simulink model "green_joint_average_motor_square_wave_harness"  (R2023b)
settings: Solver=FixedStepDiscrete  StartTime=0.0  StopTime=GJDT_StopTime  FixedStep=GJDT_TsPlant  RelTol=1e-3
values from neighbouring files (symbols this model uses):
  GJDT_IdRef_A = single(0.0)    [setup_green_joint_current_loop_twin.m]
  GJDT_Ts = 50e-6    (= 5e-05)    [setup_green_joint_current_loop_twin.m]
  GJDT_TsPlant = 5e-6    (= 5e-06)    [setup_green_joint_current_loop_twin.m]
  GJDT_Vbus_V = single(12.0)    [setup_green_joint_current_loop_twin.m]
  motor = evalin('base', 'motor')    [sweep_green_joint_speed_loop_100us_pll_candidates.m]
  simcfg = build_sim_config(cfg, module_1620)    [design_green_joint_current_loop_with_delay.m]
undefined symbols (not defined in the file or in its folder): CurDKi, CurDKp, CurQKi, CurQKp, inverter, PiCorrectionGain, VoltageEpsilon, VoltageLimitRatio
libraries: mcbplantlib x1, autolibpmsmexterior x1
Description:
  | Visible 1 kHz current-square harness. TestSupervisor is simulation-only and is not generated controller code.
settings Model: DataDictionary=green_joint_average_motor_twin_interface.sldd  Creator=user  LastModifiedBy=user
settings DebuggingCC: ParameterPrecisionLossMsg=none

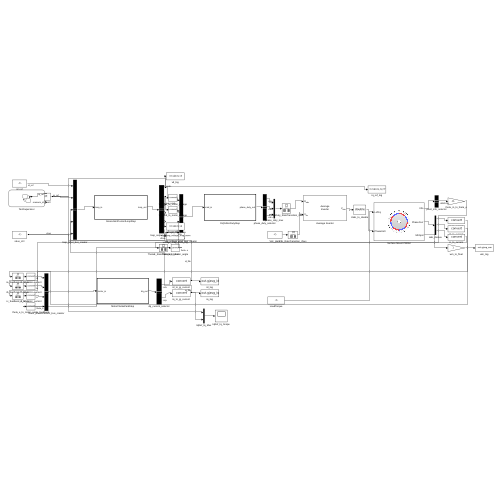
[thumbnail: Simulink's stored preview of the top-level diagram]
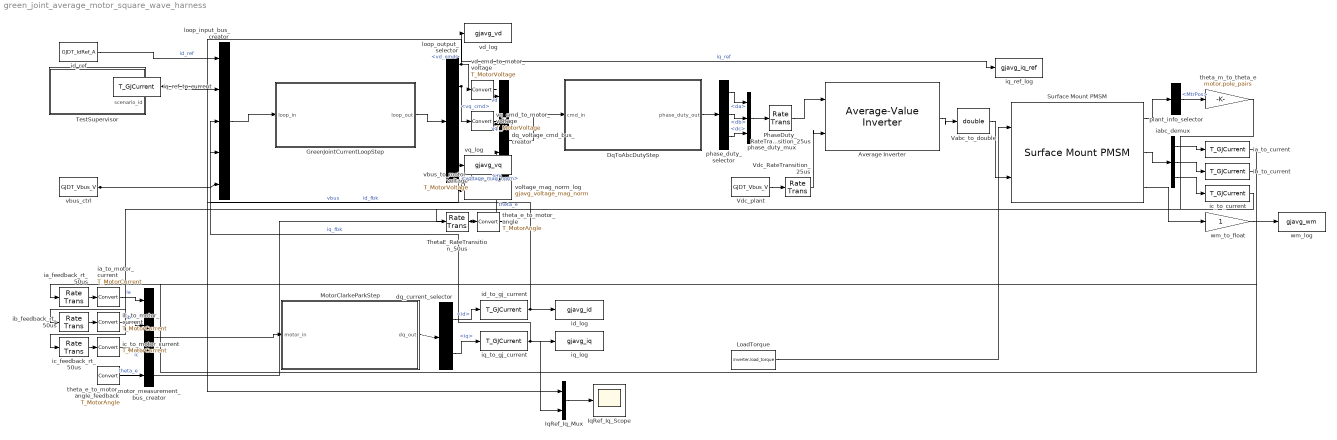
== system green_joint_average_motor_square_wave_harness ==
  Average Inverter : mcbplantlib/Average-Value Inverter
  DqToAbcDutyStep : Subsystem  TreatAsAtomicUnit=on  RTWFcnName=DqToAbcDutyStep  RTWFileName=DqToAbcDutyStep
      settings: RTWFcnNameOpts=User specified  RTWFileNameOpts=User specified
  GreenJointCurrentLoopStep : Subsystem  TreatAsAtomicUnit=on  RTWFcnName=GreenJointCurrentLoopStep  RTWFileName=GreenJointCurrentLoopStep
      settings: RTWFcnNameOpts=User specified  RTWFileNameOpts=User specified
  IqRef_Iq_Mux : Mux  Inputs=2
  IqRef_Iq_Scope : Scope
  LoadTorque : Constant  Value=inverter.load_torque  OutDataTypeStr=double  SampleTime=GJDT_TsPlant
  MotorClarkeParkStep : Subsystem  TreatAsAtomicUnit=on  RTWFcnName=MotorClarkeParkStep  RTWFileName=MotorClarkeParkStep
      settings: RTWFcnNameOpts=User specified  RTWFileNameOpts=User specified
  PhaseDuty_RateTransition_25us : RateTransition  OutPortSampleTime=GJDT_TsPlant
  Surface Mount PMSM : autolibpmsmexterior/Surface Mount PMSM  port_config=Torque  sim_type=Discrete  Ts=GJDT_TsPlant  P=motor.pole_pairs  Rs=motor.Rs  Ldq_=motor.Ld  KConstText=Permanent flux linkage constant (lambda_pm):  lambda_pm=motor.psi_f  Ke=159.9771  Kt=1.323  mechanical=[motor.J, motor.B, 0]  idq0=[0 0]  theta_init=0  omega_init=0  KConst=motor.psi_f  lambda_pm_calc=motor.psi_f  RefBlkName='autolibpmsmexterior/Surface Mount PMSM'  aMode=5  Ldq="[0.0017      0.0017]"
  TestSupervisor : Stateflow chart  TreatAsAtomicUnit=on
  ThetaE_RateTransition_50us : RateTransition  OutPortSampleTime=GJDT_Ts
  Vabc_to_double : DataTypeConversion  OutDataTypeStr=double  SaturateOnIntegerOverflow=off  RndMeth=Floor
  Vdc_RateTransition_25us : RateTransition  OutPortSampleTime=GJDT_TsPlant
  Vdc_plant : Constant  Value=GJDT_Vbus_V  OutDataTypeStr=T_GJVoltage  SampleTime=GJDT_TsPlant
  dq_current_selector : BusSelector  OutputSignals=id,iq
  dq_voltage_cmd_bus_creator : BusCreator  Inputs=4  OutDataTypeStr=Bus: open_loop_cmd_t  NonVirtualBus=on
  ia_feedback_rt_50us : RateTransition  OutPortSampleTime=GJDT_Ts
  ia_to_current : DataTypeConversion  OutDataTypeStr=T_GJCurrent  SaturateOnIntegerOverflow=off  RndMeth=Floor
  ia_to_motor_current : DataTypeConversion  OutDataTypeStr=T_MotorCurrent  SaturateOnIntegerOverflow=off  RndMeth=Floor
  iabc_demux : Demux  Outputs=3
  ib_feedback_rt_50us : RateTransition  OutPortSampleTime=GJDT_Ts
  ib_to_current : DataTypeConversion  OutDataTypeStr=T_GJCurrent  SaturateOnIntegerOverflow=off  RndMeth=Floor
  ib_to_motor_current : DataTypeConversion  OutDataTypeStr=T_MotorCurrent  SaturateOnIntegerOverflow=off  RndMeth=Floor
  ic_feedback_rt_50us : RateTransition  OutPortSampleTime=GJDT_Ts
  ic_to_current : DataTypeConversion  OutDataTypeStr=T_GJCurrent  SaturateOnIntegerOverflow=off  RndMeth=Floor
  ic_to_motor_current : DataTypeConversion  OutDataTypeStr=T_MotorCurrent  SaturateOnIntegerOverflow=off  RndMeth=Floor
  id_log : ToWorkspace  VariableName=gjavg_id  SaveFormat=Structure With Time  SampleTime=-1
  id_ref : Constant  Value=GJDT_IdRef_A  OutDataTypeStr=T_GJCurrent  SampleTime=GJDT_Ts
  id_to_gj_current : DataTypeConversion  OutDataTypeStr=T_GJCurrent  SaturateOnIntegerOverflow=off  RndMeth=Floor
  iq_log : ToWorkspace  VariableName=gjavg_iq  SaveFormat=Structure With Time  SampleTime=-1
  iq_ref_log : ToWorkspace  VariableName=gjavg_iq_ref  SaveFormat=Structure With Time  SampleTime=-1
  iq_ref_to_current : DataTypeConversion  OutDataTypeStr=T_GJCurrent  SaturateOnIntegerOverflow=off  RndMeth=Floor
  iq_to_gj_current : DataTypeConversion  OutDataTypeStr=T_GJCurrent  SaturateOnIntegerOverflow=off  RndMeth=Floor
  loop_input_bus_creator : BusCreator  Inputs=5  OutDataTypeStr=Bus: green_joint_current_loop_input_t  NonVirtualBus=on
  loop_output_selector : BusSelector  OutputSignals=vd_cmd,vq_cmd,voltage_mag,vd_norm,vq_norm,voltage_mag_norm
  motor_measurement_bus_creator : BusCreator  Inputs=4  OutDataTypeStr=Bus: motor_t  NonVirtualBus=on
  phase_duty_mux : Mux  Inputs=3
  phase_duty_selector : BusSelector  OutputSignals=da,db,dc
  plant_info_selector : BusSelector  OutputSignals=MtrPos
  theta_e_to_motor_angle : DataTypeConversion  OutDataTypeStr=T_MotorAngle  SaturateOnIntegerOverflow=off  RndMeth=Floor
  theta_e_to_motor_angle_feedback : DataTypeConversion  OutDataTypeStr=T_MotorAngle  SaturateOnIntegerOverflow=off  RndMeth=Floor
  theta_m_to_theta_e : Gain  Gain=motor.pole_pairs  OutDataTypeStr=T_GJFloat
  vbus_ctrl : Constant  Value=GJDT_Vbus_V  OutDataTypeStr=T_GJVoltage  SampleTime=GJDT_Ts
  vbus_to_motor_voltage : DataTypeConversion  OutDataTypeStr=T_MotorVoltage  SaturateOnIntegerOverflow=off  RndMeth=Floor
  vd_cmd_to_motor_voltage : DataTypeConversion  OutDataTypeStr=T_MotorVoltage  SaturateOnIntegerOverflow=off  RndMeth=Floor
  vd_log : ToWorkspace  VariableName=gjavg_vd  SaveFormat=Structure With Time  SampleTime=-1
  voltage_mag_norm_log : ToWorkspace  VariableName=gjavg_voltage_mag_norm  SaveFormat=Structure With Time  SampleTime=-1
  vq_cmd_to_motor_voltage : DataTypeConversion  OutDataTypeStr=T_MotorVoltage  SaturateOnIntegerOverflow=off  RndMeth=Floor
  vq_log : ToWorkspace  VariableName=gjavg_vq  SaveFormat=Structure With Time  SampleTime=-1
  wm_log : ToWorkspace  VariableName=gjavg_wm  SaveFormat=Structure With Time  SampleTime=-1
  wm_to_float : Gain  OutDataTypeStr=T_GJFloat
  wires:
  id_ref/1 -> loop_input_bus_creator/1  "id_ref"
  iq_ref_to_current/1 -> loop_input_bus_creator/2, iq_ref_log/1, IqRef_Iq_Mux/1  "iq_ref"
  id_to_gj_current/1 -> loop_input_bus_creator/3, id_log/1  "id_fbk"
  iq_to_gj_current/1 -> loop_input_bus_creator/4, iq_log/1, IqRef_Iq_Mux/2  "iq_fbk"
  vbus_ctrl/1 -> loop_input_bus_creator/5, vbus_to_motor_voltage/1  "vbus"
  loop_input_bus_creator/1 -> GreenJointCurrentLoopStep/1(loop_in)
  GreenJointCurrentLoopStep/1(loop_out) -> loop_output_selector/1
  loop_output_selector/1 -> vd_cmd_to_motor_voltage/1, vd_log/1  "<vd_cmd>"
  loop_output_selector/2 -> vq_cmd_to_motor_voltage/1, vq_log/1  "<vq_cmd>"
  ThetaE_RateTransition_50us/1 -> theta_e_to_motor_angle/1, theta_e_to_motor_angle_feedback/1
  vd_cmd_to_motor_voltage/1 -> dq_voltage_cmd_bus_creator/1  "vd"
  vq_cmd_to_motor_voltage/1 -> dq_voltage_cmd_bus_creator/2  "vq"
  theta_e_to_motor_angle/1 -> dq_voltage_cmd_bus_creator/3  "theta_e"
  vbus_to_motor_voltage/1 -> dq_voltage_cmd_bus_creator/4  "vdc"
  dq_voltage_cmd_bus_creator/1 -> DqToAbcDutyStep/1(cmd_in)
  DqToAbcDutyStep/1(phase_duty_out) -> phase_duty_selector/1
  phase_duty_selector/1 -> phase_duty_mux/1  "<da>"
  phase_duty_selector/2 -> phase_duty_mux/2  "<db>"
  phase_duty_selector/3 -> phase_duty_mux/3  "<dc>"
  phase_duty_mux/1 -> PhaseDuty_RateTransition_25us/1
  PhaseDuty_RateTransition_25us/1 -> Average Inverter/1
  Vdc_plant/1 -> Vdc_RateTransition_25us/1
  Vdc_RateTransition_25us/1 -> Average Inverter/2
  Average Inverter/1 -> Vabc_to_double/1
  Vabc_to_double/1 -> Surface Mount PMSM/2
  LoadTorque/1 -> Surface Mount PMSM/1
  Surface Mount PMSM/1 -> plant_info_selector/1
  plant_info_selector/1 -> theta_m_to_theta_e/1  "<MtrPos>"
  theta_m_to_theta_e/1 -> ThetaE_RateTransition_50us/1
  Surface Mount PMSM/2 -> iabc_demux/1
  iabc_demux/1 -> ia_to_current/1
  iabc_demux/2 -> ib_to_current/1
  iabc_demux/3 -> ic_to_current/1
  ia_to_current/1 -> ia_feedback_rt_50us/1
  ib_to_current/1 -> ib_feedback_rt_50us/1
  ic_to_current/1 -> ic_feedback_rt_50us/1
  ia_feedback_rt_50us/1 -> ia_to_motor_current/1
  ib_feedback_rt_50us/1 -> ib_to_motor_current/1
  ic_feedback_rt_50us/1 -> ic_to_motor_current/1
  ia_to_motor_current/1 -> motor_measurement_bus_creator/1  "ia"
  ib_to_motor_current/1 -> motor_measurement_bus_creator/2  "ib"
  ic_to_motor_current/1 -> motor_measurement_bus_creator/3  "ic"
  theta_e_to_motor_angle_feedback/1 -> motor_measurement_bus_creator/4  "theta_e"
  motor_measurement_bus_creator/1 -> MotorClarkeParkStep/1(motor_in)
  MotorClarkeParkStep/1(dq_out) -> dq_current_selector/1
  dq_current_selector/1 -> id_to_gj_current/1  "<id>"
  dq_current_selector/2 -> iq_to_gj_current/1  "<iq>"
  loop_output_selector/6 -> voltage_mag_norm_log/1  "<voltage_mag_norm>"
  Surface Mount PMSM/3 -> wm_to_float/1
  wm_to_float/1 -> wm_log/1
  TestSupervisor/1(iq_ref) -> iq_ref_to_current/1
  IqRef_Iq_Mux/1 -> IqRef_Iq_Scope/1

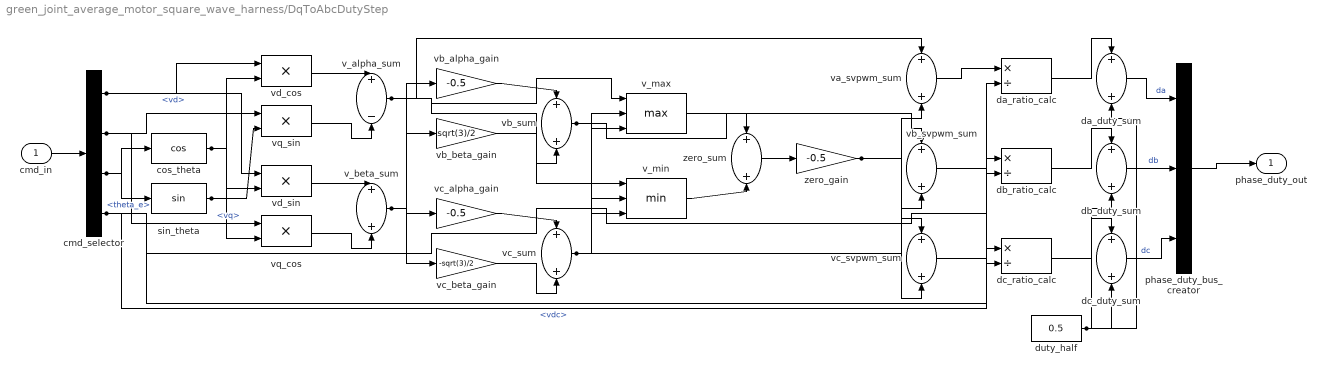
== system green_joint_average_motor_square_wave_harness/DqToAbcDutyStep ==
  cmd_in : Inport  OutDataTypeStr=Bus: open_loop_cmd_t  BusOutputAsStruct=on
  cmd_selector : BusSelector  OutputSignals=vd,vq,theta_e,vdc
  cos_theta : Trigonometry  Operator=cos
  da_duty_sum : Sum  OutDataTypeStr=T_DutyRatio  AccumDataTypeStr=T_DutyRatio
  da_ratio_calc : Product  Inputs=*/  OutDataTypeStr=T_DutyRatio
  db_duty_sum : Sum  OutDataTypeStr=T_DutyRatio  AccumDataTypeStr=T_DutyRatio
  db_ratio_calc : Product  Inputs=*/  OutDataTypeStr=T_DutyRatio
  dc_duty_sum : Sum  OutDataTypeStr=T_DutyRatio  AccumDataTypeStr=T_DutyRatio
  dc_ratio_calc : Product  Inputs=*/  OutDataTypeStr=T_DutyRatio
  duty_half : Constant  Value=0.5  OutDataTypeStr=T_DutyRatio  SampleTime=simcfg.Ts_ctrl
  phase_duty_bus_creator : BusCreator  Inputs=3  OutDataTypeStr=Bus: phase_duty_t  NonVirtualBus=on
  sin_theta : Trigonometry
  v_alpha_sum : Sum  Inputs=+-  OutDataTypeStr=T_MotorVoltage  AccumDataTypeStr=T_MotorVoltage
  v_beta_sum : Sum  OutDataTypeStr=T_MotorVoltage  AccumDataTypeStr=T_MotorVoltage
  v_max : MinMax  Function=max  Inputs=3
  v_min : MinMax  Inputs=3
  va_svpwm_sum : Sum  OutDataTypeStr=T_MotorVoltage  AccumDataTypeStr=T_MotorVoltage
  vb_alpha_gain : Gain  Gain=-0.5  ParamDataTypeStr=T_MotorFloat  OutDataTypeStr=T_MotorVoltage
  vb_beta_gain : Gain  Gain=sqrt(3)/2  ParamDataTypeStr=T_MotorFloat  OutDataTypeStr=T_MotorVoltage
  vb_sum : Sum  OutDataTypeStr=T_MotorVoltage  AccumDataTypeStr=T_MotorVoltage
  vb_svpwm_sum : Sum  OutDataTypeStr=T_MotorVoltage  AccumDataTypeStr=T_MotorVoltage
  vc_alpha_gain : Gain  Gain=-0.5  ParamDataTypeStr=T_MotorFloat  OutDataTypeStr=T_MotorVoltage
  vc_beta_gain : Gain  Gain=-sqrt(3)/2  ParamDataTypeStr=T_MotorFloat  OutDataTypeStr=T_MotorVoltage
  vc_sum : Sum  OutDataTypeStr=T_MotorVoltage  AccumDataTypeStr=T_MotorVoltage
  vc_svpwm_sum : Sum  OutDataTypeStr=T_MotorVoltage  AccumDataTypeStr=T_MotorVoltage
  vd_cos : Product  Inputs=**  OutDataTypeStr=T_MotorVoltage
  vd_sin : Product  Inputs=**  OutDataTypeStr=T_MotorVoltage
  vq_cos : Product  Inputs=**  OutDataTypeStr=T_MotorVoltage
  vq_sin : Product  Inputs=**  OutDataTypeStr=T_MotorVoltage
  zero_gain : Gain  Gain=-0.5  ParamDataTypeStr=T_MotorFloat  OutDataTypeStr=T_MotorVoltage
  zero_sum : Sum  OutDataTypeStr=T_MotorVoltage  AccumDataTypeStr=T_MotorVoltage
  phase_duty_out : Outport  OutDataTypeStr=Bus: phase_duty_t
  wires:
  phase_duty_bus_creator/1 -> phase_duty_out/1
  dc_duty_sum/1 -> phase_duty_bus_creator/3  "dc"
  db_duty_sum/1 -> phase_duty_bus_creator/2  "db"
  da_duty_sum/1 -> phase_duty_bus_creator/1  "da"
  duty_half/1 -> dc_duty_sum/2, db_duty_sum/2, da_duty_sum/2
  dc_ratio_calc/1 -> dc_duty_sum/1
  db_ratio_calc/1 -> db_duty_sum/1
  da_ratio_calc/1 -> da_duty_sum/1
  vc_svpwm_sum/1 -> dc_ratio_calc/1
  vb_svpwm_sum/1 -> db_ratio_calc/1
  cmd_selector/4 -> dc_ratio_calc/2, db_ratio_calc/2, da_ratio_calc/2  "<vdc>"
  va_svpwm_sum/1 -> da_ratio_calc/1
  zero_gain/1 -> vc_svpwm_sum/2, vb_svpwm_sum/2, va_svpwm_sum/2
  zero_sum/1 -> zero_gain/1
  v_min/1 -> zero_sum/2
  v_max/1 -> zero_sum/1
  vc_sum/1 -> vc_svpwm_sum/1, v_min/3, v_max/3
  vb_sum/1 -> vb_svpwm_sum/1, v_min/2, v_max/2
  vc_beta_gain/1 -> vc_sum/2
  vc_alpha_gain/1 -> vc_sum/1
  vb_beta_gain/1 -> vb_sum/2
  vb_alpha_gain/1 -> vb_sum/1
  v_beta_sum/1 -> vc_beta_gain/1, vb_beta_gain/1
  v_alpha_sum/1 -> va_svpwm_sum/1, v_min/1, v_max/1, vc_alpha_gain/1, vb_alpha_gain/1
  vq_cos/1 -> v_beta_sum/2
  vd_sin/1 -> v_beta_sum/1
  vq_sin/1 -> v_alpha_sum/2
  vd_cos/1 -> v_alpha_sum/1
  sin_theta/1 -> vd_sin/2, vq_sin/2
  cmd_selector/2 -> vq_cos/1, vq_sin/1  "<vq>"
  cos_theta/1 -> vq_cos/2, vd_cos/2
  cmd_selector/1 -> vd_sin/1, vd_cos/1  "<vd>"
  cmd_selector/3 -> sin_theta/1, cos_theta/1  "<theta_e>"
  cmd_in/1 -> cmd_selector/1

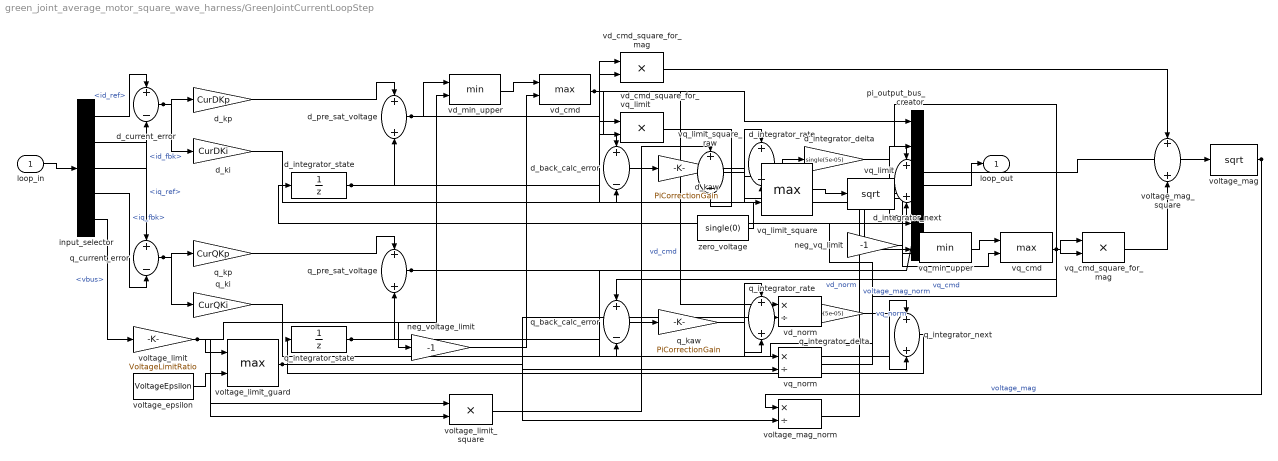
== system green_joint_average_motor_square_wave_harness/GreenJointCurrentLoopStep ==
  loop_in : Inport  OutDataTypeStr=Bus: green_joint_current_loop_input_t  BusOutputAsStruct=on
  d_back_calc_error : Sum  Inputs=+-  OutDataTypeStr=T_GJVoltage  AccumDataTypeStr=T_GJVoltage
  d_current_error : Sum  Inputs=+-  OutDataTypeStr=T_GJCurrent  AccumDataTypeStr=T_GJCurrent
  d_integrator_delta : Gain  Gain=single(5e-05)  ParamDataTypeStr=T_GJFloat  OutDataTypeStr=T_GJVoltage
  d_integrator_next : Sum  OutDataTypeStr=T_GJVoltage  AccumDataTypeStr=T_GJVoltage
  d_integrator_rate : Sum  OutDataTypeStr=T_GJVoltage  AccumDataTypeStr=T_GJVoltage
  d_integrator_state : UnitDelay  InitialCondition=single(0)  SampleTime=5e-05  HasFrameUpgradeWarning=on
  d_kaw : Gain  Gain=PiCorrectionGain  ParamDataTypeStr=T_GJFloat  OutDataTypeStr=T_GJVoltage
  d_ki : Gain  Gain=CurDKi  ParamDataTypeStr=T_GJFloat  OutDataTypeStr=T_GJVoltage
  d_kp : Gain  Gain=CurDKp  ParamDataTypeStr=T_GJFloat  OutDataTypeStr=T_GJVoltage
  d_pre_sat_voltage : Sum  OutDataTypeStr=T_GJVoltage  AccumDataTypeStr=T_GJVoltage
  input_selector : BusSelector  OutputSignals=id_ref,iq_ref,id_fbk,iq_fbk,vbus
  neg_voltage_limit : Gain  Gain=-1  ParamDataTypeStr=T_GJFloat  OutDataTypeStr=T_GJVoltage
  neg_vq_limit : Gain  Gain=-1  ParamDataTypeStr=T_GJFloat  OutDataTypeStr=T_GJVoltage
  pi_output_bus_creator : BusCreator  Inputs=6  OutDataTypeStr=Bus: green_joint_current_loop_output_t  NonVirtualBus=on
  q_back_calc_error : Sum  Inputs=+-  OutDataTypeStr=T_GJVoltage  AccumDataTypeStr=T_GJVoltage
  q_current_error : Sum  Inputs=+-  OutDataTypeStr=T_GJCurrent  AccumDataTypeStr=T_GJCurrent
  q_integrator_delta : Gain  Gain=single(5e-05)  ParamDataTypeStr=T_GJFloat  OutDataTypeStr=T_GJVoltage
  q_integrator_next : Sum  OutDataTypeStr=T_GJVoltage  AccumDataTypeStr=T_GJVoltage
  q_integrator_rate : Sum  OutDataTypeStr=T_GJVoltage  AccumDataTypeStr=T_GJVoltage
  q_integrator_state : UnitDelay  InitialCondition=single(0)  SampleTime=5e-05  HasFrameUpgradeWarning=on
  q_kaw : Gain  Gain=PiCorrectionGain  ParamDataTypeStr=T_GJFloat  OutDataTypeStr=T_GJVoltage
  q_ki : Gain  Gain=CurQKi  ParamDataTypeStr=T_GJFloat  OutDataTypeStr=T_GJVoltage
  q_kp : Gain  Gain=CurQKp  ParamDataTypeStr=T_GJFloat  OutDataTypeStr=T_GJVoltage
  q_pre_sat_voltage : Sum  OutDataTypeStr=T_GJVoltage  AccumDataTypeStr=T_GJVoltage
  vd_cmd : MinMax  Function=max  Inputs=2
  vd_cmd_square_for_mag : Product  Inputs=**  OutDataTypeStr=T_GJVoltage
  vd_cmd_square_for_vq_limit : Product  Inputs=**  OutDataTypeStr=T_GJVoltage
  vd_min_upper : MinMax  Inputs=2
  vd_norm : Product  Inputs=*/  OutDataTypeStr=T_GJVoltageNorm
  voltage_epsilon : Constant  Value=VoltageEpsilon  OutDataTypeStr=T_GJVoltage  SampleTime=-1
  voltage_limit : Gain  Gain=VoltageLimitRatio  ParamDataTypeStr=T_GJFloat  OutDataTypeStr=T_GJVoltage
  voltage_limit_guard : MinMax  Function=max  Inputs=2
  voltage_limit_square : Product  Inputs=**  OutDataTypeStr=T_GJVoltage
  voltage_mag : Math  Operator=sqrt  OutDataTypeStr=T_GJVoltage
  voltage_mag_norm : Product  Inputs=*/  OutDataTypeStr=T_GJVoltageNorm
  voltage_mag_square : Sum  OutDataTypeStr=T_GJVoltage  AccumDataTypeStr=T_GJVoltage
  vq_cmd : MinMax  Function=max  Inputs=2
  vq_cmd_square_for_mag : Product  Inputs=**  OutDataTypeStr=T_GJVoltage
  vq_limit : Math  Operator=sqrt  OutDataTypeStr=T_GJVoltage
  vq_limit_square : MinMax  Function=max  Inputs=2
  vq_limit_square_raw : Sum  Inputs=+-  OutDataTypeStr=T_GJVoltage  AccumDataTypeStr=T_GJVoltage
  vq_min_upper : MinMax  Inputs=2
  vq_norm : Product  Inputs=*/  OutDataTypeStr=T_GJVoltageNorm
  zero_voltage : Constant  Value=single(0)  OutDataTypeStr=T_GJVoltage  SampleTime=-1
  loop_out : Outport  OutDataTypeStr=Bus: green_joint_current_loop_output_t
  wires:
  pi_output_bus_creator/1 -> loop_out/1
  voltage_mag_norm/1 -> pi_output_bus_creator/6  "voltage_mag_norm"
  vq_norm/1 -> pi_output_bus_creator/5  "vq_norm"
  vd_norm/1 -> pi_output_bus_creator/4  "vd_norm"
  voltage_mag/1 -> pi_output_bus_creator/3, voltage_mag_norm/1  "voltage_mag"
  voltage_limit_guard/1 -> voltage_mag_norm/2, vq_norm/2, vd_norm/2
  voltage_mag_square/1 -> voltage_mag/1
  vq_cmd_square_for_mag/1 -> voltage_mag_square/2
  vd_cmd_square_for_mag/1 -> voltage_mag_square/1
  vq_cmd/1 -> pi_output_bus_creator/2, vq_norm/1, q_back_calc_error/1, vq_cmd_square_for_mag/2, vq_cmd_square_for_mag/1  "vq_cmd"
  neg_vq_limit/1 -> vq_cmd/2
  vq_min_upper/1 -> vq_cmd/1
  q_pre_sat_voltage/1 -> q_back_calc_error/2, vq_min_upper/1
  vq_limit/1 -> vq_min_upper/2, neg_vq_limit/1
  vq_limit_square/1 -> vq_limit/1
  zero_voltage/1 -> vq_limit_square/2
  vq_limit_square_raw/1 -> vq_limit_square/1
  vd_cmd_square_for_vq_limit/1 -> vq_limit_square_raw/2
  voltage_limit_square/1 -> vq_limit_square_raw/1
  vd_cmd/1 -> pi_output_bus_creator/1, vd_norm/1, d_back_calc_error/1, vd_cmd_square_for_mag/2, vd_cmd_square_for_mag/1, vd_cmd_square_for_vq_limit/2, vd_cmd_square_for_vq_limit/1  "vd_cmd"
  neg_voltage_limit/1 -> vd_cmd/2
  vd_min_upper/1 -> vd_cmd/1
  d_pre_sat_voltage/1 -> d_back_calc_error/2, vd_min_upper/1
  q_integrator_next/1 -> q_integrator_state/1
  q_integrator_delta/1 -> q_integrator_next/2
  q_integrator_rate/1 -> q_integrator_delta/1
  q_kaw/1 -> q_integrator_rate/2
  q_back_calc_error/1 -> q_kaw/1
  q_ki/1 -> q_integrator_rate/1
  q_integrator_state/1 -> q_integrator_next/1, q_pre_sat_voltage/2
  q_kp/1 -> q_pre_sat_voltage/1
  q_current_error/1 -> q_ki/1, q_kp/1
  input_selector/4 -> q_current_error/2  "<iq_fbk>"
  input_selector/2 -> q_current_error/1  "<iq_ref>"
  d_integrator_next/1 -> d_integrator_state/1
  d_integrator_delta/1 -> d_integrator_next/2
  d_integrator_rate/1 -> d_integrator_delta/1
  d_kaw/1 -> d_integrator_rate/2
  d_back_calc_error/1 -> d_kaw/1
  d_ki/1 -> d_integrator_rate/1
  d_integrator_state/1 -> d_integrator_next/1, d_pre_sat_voltage/2
  d_kp/1 -> d_pre_sat_voltage/1
  d_current_error/1 -> d_ki/1, d_kp/1
  input_selector/3 -> d_current_error/2  "<id_fbk>"
  input_selector/1 -> d_current_error/1  "<id_ref>"
  voltage_epsilon/1 -> voltage_limit_guard/2
  voltage_limit/1 -> voltage_limit_square/2, voltage_limit_square/1, vd_min_upper/2, neg_voltage_limit/1, voltage_limit_guard/1
  input_selector/5 -> voltage_limit/1  "<vbus>"
  loop_in/1 -> input_selector/1

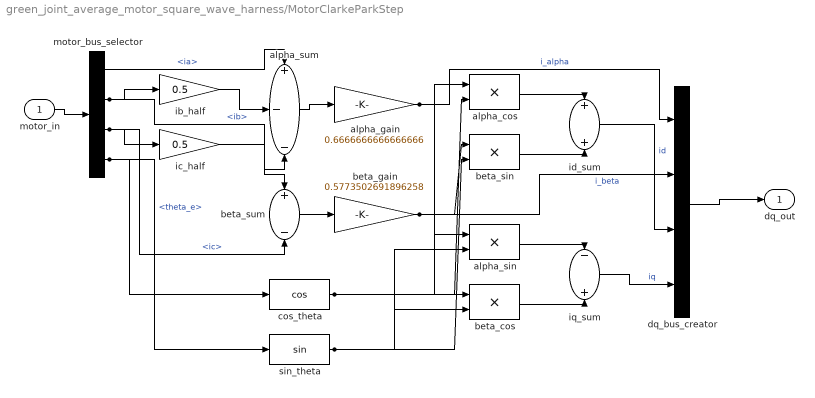
== system green_joint_average_motor_square_wave_harness/MotorClarkeParkStep ==
  motor_in : Inport  OutDataTypeStr=Bus: motor_t  BusOutputAsStruct=on
  alpha_cos : Product  Inputs=**  OutDataTypeStr=T_MotorCurrent  SaturateOnIntegerOverflow=on
  alpha_gain : Gain  Gain=0.6666666666666666  ParamDataTypeStr=T_MotorCurrent  OutDataTypeStr=T_MotorCurrent  SaturateOnIntegerOverflow=on
  alpha_sin : Product  Inputs=**  OutDataTypeStr=T_MotorCurrent  SaturateOnIntegerOverflow=on
  alpha_sum : Sum  Inputs=+--  OutDataTypeStr=T_MotorCurrent  AccumDataTypeStr=T_MotorCurrent  SaturateOnIntegerOverflow=on
  beta_cos : Product  Inputs=**  OutDataTypeStr=T_MotorCurrent  SaturateOnIntegerOverflow=on
  beta_gain : Gain  Gain=0.5773502691896258  ParamDataTypeStr=T_MotorCurrent  OutDataTypeStr=T_MotorCurrent  SaturateOnIntegerOverflow=on
  beta_sin : Product  Inputs=**  OutDataTypeStr=T_MotorCurrent  SaturateOnIntegerOverflow=on
  beta_sum : Sum  Inputs=+-  OutDataTypeStr=T_MotorCurrent  AccumDataTypeStr=T_MotorCurrent  SaturateOnIntegerOverflow=on
  cos_theta : Trigonometry  Operator=cos
  dq_bus_creator : BusCreator  Inputs=4  OutDataTypeStr=Bus: motor_dq_t  NonVirtualBus=on
  ib_half : Gain  Gain=0.5  ParamDataTypeStr=T_MotorCurrent  OutDataTypeStr=T_MotorCurrent  SaturateOnIntegerOverflow=on
  ic_half : Gain  Gain=0.5  ParamDataTypeStr=T_MotorCurrent  OutDataTypeStr=T_MotorCurrent  SaturateOnIntegerOverflow=on
  id_sum : Sum  OutDataTypeStr=T_MotorCurrent  AccumDataTypeStr=T_MotorCurrent  SaturateOnIntegerOverflow=on
  iq_sum : Sum  Inputs=-+  OutDataTypeStr=T_MotorCurrent  AccumDataTypeStr=T_MotorCurrent  SaturateOnIntegerOverflow=on
  motor_bus_selector : BusSelector  OutputSignals=ia,ib,ic,theta_e
  sin_theta : Trigonometry
  dq_out : Outport  OutDataTypeStr=Bus: motor_dq_t
  wires:
  dq_bus_creator/1 -> dq_out/1
  iq_sum/1 -> dq_bus_creator/4  "iq"
  id_sum/1 -> dq_bus_creator/3  "id"
  beta_cos/1 -> iq_sum/2
  alpha_sin/1 -> iq_sum/1
  beta_sin/1 -> id_sum/2
  alpha_cos/1 -> id_sum/1
  sin_theta/1 -> alpha_sin/2, beta_sin/2
  beta_gain/1 -> dq_bus_creator/2, beta_cos/1, beta_sin/1  "i_beta"
  cos_theta/1 -> beta_cos/2, alpha_cos/2
  alpha_gain/1 -> dq_bus_creator/1, alpha_sin/1, alpha_cos/1  "i_alpha"
  motor_bus_selector/4 -> sin_theta/1, cos_theta/1  "<theta_e>"
  beta_sum/1 -> beta_gain/1
  alpha_sum/1 -> alpha_gain/1
  ic_half/1 -> alpha_sum/3
  ib_half/1 -> alpha_sum/2
  motor_bus_selector/3 -> beta_sum/2, ic_half/1  "<ic>"
  motor_bus_selector/2 -> beta_sum/1, ib_half/1  "<ib>"
  motor_bus_selector/1 -> alpha_sum/1  "<ia>"
  motor_in/1 -> motor_bus_selector/1

== stateflow chart green_joint_average_motor_square_wave_harness/TestSupervisor ==
  state CurrentSquareLow
    during:
    iq_ref = -single(0.3);
    scenario_id = int32(1);
  state CurrentSquareHigh
    during:
    iq_ref = single(0.3);
    scenario_id = int32(1);
  (default) -> CurrentSquareLow
  CurrentSquareHigh -> CurrentSquareLow : after(10,tick)
  CurrentSquareLow -> CurrentSquareHigh : after(10,tick)
  data: iq_ref output; scenario_id output
